simulink model "AMPC_OA_model"  (R2023b)
settings: Solver=FixedStepAuto  StartTime=0.0  StopTime=600  FixedStep=0.1  RelTol=1e-3
InitFcn:
  | clear
  | v_x = 0; v_h = 0;
  | ts = 0.1; m = 240; rou = 1.225; Cd = 1; Fx = 2.11; Fh = 1.47;
  | Kp1 = 416.55; Kp2 = 1559.85;
  | Ki1 = 133.89; Ki2 = 943.53;
  | Kd1 = 43.47; Kd2 = -103.95;
  | a1 = -0.5/m*rou*Cd*Fx*v_x; a2 = -0.5/m*rou*Cd*Fh*v_h;
  | b1 = 1/m; b2 = 1/m;
  | num = {[Kd1*b1 Kp1*b1 Ki1*b1] 0; 0 [Kd2*b2, Kp2*b2, Ki2*b2]};
  | den = {[Kd1*b1+1 Kp1*b1-a1 Ki1*b1 0] 1; 1 [Kd2*b2+1 Kp2*b2-a2 Ki2*b2 0]};
  | 
  | plant = ss(c2d(tf(num, den),ts));
  | MV = struct("Min",{0; -5},"Max",{30; 8},"RateMin",{-8*ts; -5*ts},"RateMax",{8*ts; 5*ts});
  | Weights = struct('MV',[10 10],'MVRate',[100 100],'Output',[1 1],"ECR",100000);
  | mpcobj =  mpc(plant,ts,20,1,Weights,MV);
  | E = [0 0]; F = [1 -1]; G = 0; S = 0;
  | setconstraint(mpcobj,E,F,G)
  | display(mpcobj)
  | display(tf(num, den))
StopFcn:
  | hold on
  | plot(out.x,out.h,LineWidth=2)
  | plot(polyshape([0 300 10000-300 10000],[0 300 300 0]))
libraries: slpidlib x2, mpclib x1, matrix_library x1
settings Model: Creator=Felix_Soong  LastModifiedBy=Felix_Soong

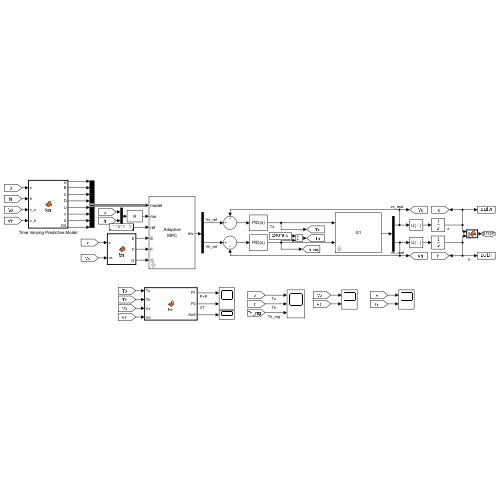
[thumbnail: Simulink's stored preview of the top-level diagram]
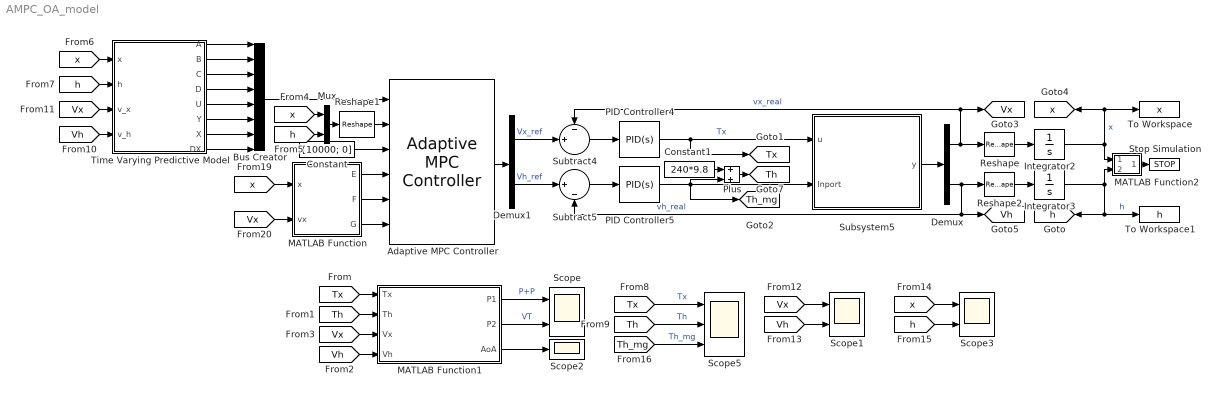
== system AMPC_OA_model ==
  Adaptive MPC Controller : mpclib/Adaptive MPC Controller  SCDEnableBlockLinearizationSpecification=on  mpcobj=mpcobj  enable_value=0  updateMPCinCallerWorkspace=on  md_inport=off  mv_inport=off  uref_inport=off  return_cost=off  return_mvseq=off  return_qpstatus=off  return_xseq=off  return_state=off  return_ovseq=off  state_inport=off  isltv_plant=off  umin_inport=off  umax_inport=off  ymin_inport=off  ymax_inport=off  cc_inport=on  ywt_inport=off  uwt_inport=off  duwt_inport=off  rhoeps_inport=off  pm_inport=off  MaximumP=10  HorizonChoice=FixedHorizon  BlockDataType=double  SampleTimeInherited=off  switch_inport=off
  Bus Creator : BusCreator  Inputs=8
  Constant : Constant  Value=[10000; 0]
  Constant1 : Constant  Value=240*9.8
  Demux : Demux  Outputs=2
  Demux1 : Demux  Outputs=2
  Integrator2 : Integrator
  Integrator3 : Integrator
  MATLAB Function : MATLAB Function  TreatAsAtomicUnit=on
  MATLAB Function1 : MATLAB Function  TreatAsAtomicUnit=on
  MATLAB Function2 : MATLAB Function  TreatAsAtomicUnit=on
  Mux : Mux  Inputs=2
  PID Controller4 : slpidlib/PID Controller  Controller=PID  Form=Parallel  TimeDomain=Continuous-time  UseExternalTs=off  SampleTime=-1  IntegratorMethod=Forward Euler  FilterMethod=Forward Euler  ControllerParametersSource=internal  P=416.552891741816  I=133.885986163438  UseKiTs=off  D=43.4731448254193  N=6.63612888550275  UseFilter=on  TunerSelectOption=Transfer Function Based (PID Tuner App)  InitialConditionSource=internal  InitialConditionForIntegrator=0  InitialConditionForFilter=0  DifferentiatorICPrevScaledInput=0  ExternalReset=none  TrackingMode=off  Kt=1  LimitOutput=off  SatLimitsSource=internal  UpperSaturationLimit=inf  LowerSaturationLimit=-inf  LinearizeAsGain=on  AntiWindupMode=none  Kb=1  LimitIntegrator=off  UpperIntegratorSaturationLimit=inf  LowerIntegratorSaturationLimit=-inf  POutMin=[]  POutMax=[]  IOutMin=[]  IOutMax=[]  DOutMin=[]  DOutMax=[]  NOutMin=[]  NOutMax=[]  SumOutMin=[]  SumOutMax=[]  SaturationOutMin=[]  SaturationOutMax=[]  PParamMin=[]  PParamMax=[]  IParamMin=[]  IParamMax=[]  DParamMin=[]  DParamMax=[]  NParamMin=[]  NParamMax=[]  KbParamMin=[]  KbParamMax=[]  KtParamMin=[]  KtParamMax=[]  KbOutMin=[]  KbOutMax=[]  KtOutMin=[]  KtOutMax=[]  IntegratorOutMin=[]  IntegratorOutMax=[]  FilterOutMin=[]  FilterOutMax=[]  SumI1OutMin=[]  SumI1OutMax=[]  SumI2OutMin=[]  SumI2OutMax=[]  SumI3OutMin=[]  SumI3OutMax=[]  SumI4OutMin=[]  SumI4OutMax=[]  SumDOutMin=[]  SumDOutMax=[]  DifferentiatorOutMin=[]  DifferentiatorOutMax=[]  FilterDiffOutCoefMin=[]  FilterDiffOutCoefMax=[]  ReciprocalOutMin=[]  ReciprocalOutMax=[]  SumDenOutMin=[]  SumDenOutMax=[]  SumNumOutMin=[]  SumNumOutMax=[]  DivideOutMin=[]  DivideOutMax=[]  UdiffTsProdOutMin=[]  UdiffTsProdOutMax=[]  NTsProdOutMin=[]  NTsProdOutMax=[]  UintegralTsProdOutMin=[]  UintegralTsProdOutMax=[]  UngainTsProdOutMin=[]  UngainTsProdOutMax=[]  ClampingZeroOutDataTypeStr=Inherit: Inherit via back propagation  ClampingZeroOutMin=[]  ClampingZeroOutMax=[]  FilterDenConstantOutDataTypeStr=Inherit: Inherit via back propagation  FilterDenConstantOutMin=[]  FilterDenConstantOutMax=[]  PCopyOutDataTypeStr=Inherit: Inherit via back propagation  PCopyOutMin=[]  PCopyOutMax=[]  NCopyOutDataTypeStr=Inherit: Inherit via back propagation  NCopyOutMin=[]  NCopyOutMax=[]  IntegratorContinuousStateAttributes=''  IntegratorStateMustResolveToSignalObject=off  IntegratorRTWStateStorageClass=Auto  FilterContinuousStateAttributes=''  FilterStateMustResolveToSignalObject=off  FilterRTWStateStorageClass=Auto  ParallelPVariant=InternalParameters  IdealPVariant=Disabled  IVariant=InternalParameters  DVariant=InternalParameters  IntegratorVariant=Continuous  SatVariant=Disabled  AWVariant=Passthrough  PCopyVariant=Disabled  TRVariant=Disabled  FdbkBlocksVariant=Forward  IdealPFdbkVariant=Disabled  SatFdbkVariant=Disabled  DerivativeFilterVariant=ContFilter  NVariant=InternalParameters  NCopyVariant=Disabled  FilterICVariant=InternalICsFilter  IntegratorICVariant=InternalICs  ExternalResetVariant=Disabled  TRSumVariant=Passthrough  SumFdbkVariant=Disabled  SumVariant=Sum_PID  TsampFilterVariant=InternalTs  TsampNgainVariant=Passthrough  TsampIntegralVariant=Disabled_SignalSpec  ExternalSaturationOutDataTypeStr=Inherit: Same as second input
  PID Controller5 : slpidlib/PID Controller  Controller=PID  Form=Parallel  TimeDomain=Continuous-time  UseExternalTs=off  SampleTime=-1  IntegratorMethod=Forward Euler  FilterMethod=Forward Euler  ControllerParametersSource=internal  P=1559.8476067563  I=943.53288128348  UseKiTs=off  D=-103.949358808692  N=5.44051767311659  UseFilter=on  TunerSelectOption=Transfer Function Based (PID Tuner App)  InitialConditionSource=internal  InitialConditionForIntegrator=0  InitialConditionForFilter=0  DifferentiatorICPrevScaledInput=0  ExternalReset=none  TrackingMode=off  Kt=1  LimitOutput=off  SatLimitsSource=internal  UpperSaturationLimit=inf  LowerSaturationLimit=-inf  LinearizeAsGain=on  AntiWindupMode=none  Kb=1  LimitIntegrator=off  UpperIntegratorSaturationLimit=inf  LowerIntegratorSaturationLimit=-inf  POutMin=[]  POutMax=[]  IOutMin=[]  IOutMax=[]  DOutMin=[]  DOutMax=[]  NOutMin=[]  NOutMax=[]  SumOutMin=[]  SumOutMax=[]  SaturationOutMin=[]  SaturationOutMax=[]  PParamMin=[]  PParamMax=[]  IParamMin=[]  IParamMax=[]  DParamMin=[]  DParamMax=[]  NParamMin=[]  NParamMax=[]  KbParamMin=[]  KbParamMax=[]  KtParamMin=[]  KtParamMax=[]  KbOutMin=[]  KbOutMax=[]  KtOutMin=[]  KtOutMax=[]  IntegratorOutMin=[]  IntegratorOutMax=[]  FilterOutMin=[]  FilterOutMax=[]  SumI1OutMin=[]  SumI1OutMax=[]  SumI2OutMin=[]  SumI2OutMax=[]  SumI3OutMin=[]  SumI3OutMax=[]  SumI4OutMin=[]  SumI4OutMax=[]  SumDOutMin=[]  SumDOutMax=[]  DifferentiatorOutMin=[]  DifferentiatorOutMax=[]  FilterDiffOutCoefMin=[]  FilterDiffOutCoefMax=[]  ReciprocalOutMin=[]  ReciprocalOutMax=[]  SumDenOutMin=[]  SumDenOutMax=[]  SumNumOutMin=[]  SumNumOutMax=[]  DivideOutMin=[]  DivideOutMax=[]  UdiffTsProdOutMin=[]  UdiffTsProdOutMax=[]  NTsProdOutMin=[]  NTsProdOutMax=[]  UintegralTsProdOutMin=[]  UintegralTsProdOutMax=[]  UngainTsProdOutMin=[]  UngainTsProdOutMax=[]  ClampingZeroOutDataTypeStr=Inherit: Inherit via back propagation  ClampingZeroOutMin=[]  ClampingZeroOutMax=[]  FilterDenConstantOutDataTypeStr=Inherit: Inherit via back propagation  FilterDenConstantOutMin=[]  FilterDenConstantOutMax=[]  PCopyOutDataTypeStr=Inherit: Inherit via back propagation  PCopyOutMin=[]  PCopyOutMax=[]  NCopyOutDataTypeStr=Inherit: Inherit via back propagation  NCopyOutMin=[]  NCopyOutMax=[]  IntegratorContinuousStateAttributes=''  IntegratorStateMustResolveToSignalObject=off  IntegratorRTWStateStorageClass=Auto  FilterContinuousStateAttributes=''  FilterStateMustResolveToSignalObject=off  FilterRTWStateStorageClass=Auto  ParallelPVariant=InternalParameters  IdealPVariant=Disabled  IVariant=InternalParameters  DVariant=InternalParameters  IntegratorVariant=Continuous  SatVariant=Disabled  AWVariant=Passthrough  PCopyVariant=Disabled  TRVariant=Disabled  FdbkBlocksVariant=Forward  IdealPFdbkVariant=Disabled  SatFdbkVariant=Disabled  DerivativeFilterVariant=ContFilter  NVariant=InternalParameters  NCopyVariant=Disabled  FilterICVariant=InternalICsFilter  IntegratorICVariant=InternalICs  ExternalResetVariant=Disabled  TRSumVariant=Passthrough  SumFdbkVariant=Disabled  SumVariant=Sum_PID  TsampFilterVariant=InternalTs  TsampNgainVariant=Passthrough  TsampIntegralVariant=Disabled_SignalSpec  ExternalSaturationOutDataTypeStr=Inherit: Same as second input
  Plus : Sum
  Reshape : Reshape
  Reshape1 : Reshape  OutputDimensionality=Customize  OutputDimensions=[2,1]
  Reshape2 : Reshape
  Scope : Scope  NumInputPorts=2
  Scope1 : Scope  NumInputPorts=2
  Scope2 : Scope
  Scope3 : Scope  NumInputPorts=2
  Scope5 : Scope  NumInputPorts=3
  Stop Simulation : Stop
  Subsystem5 : Subsystem  mask{m=240, Fx=2.11, Fh=1.47, Cd=1, rou=1.225}
      mask prompts: m "mass"; rou "air density"
      mask DialogControl ParameterGroupVar Prompt: 参数
      mask Display: disp('G1');
  Subtract4 : Sum  Inputs=-|+||
  Subtract5 : Sum  Inputs=||+|-
  Time Varying Predictive Model : MATLAB Function  TreatAsAtomicUnit=on
  To Workspace : ToWorkspace  VariableName=x  SampleTime=-1
  To Workspace1 : ToWorkspace  VariableName=h  SampleTime=-1
  tag scope: Th=global, Th_mg=global, Tx=global, Vh=global, Vx=global, h=global, x=global
  wires:
  Subtract5/1 -> PID Controller5/1
  Subtract4/1 -> PID Controller4/1
  Subsystem5/1(y) -> Demux/1
  Demux/1 -> Subtract4/1, [Vx], Reshape/1  "vx_real"
  Demux/2 -> Reshape2/1, [Vh], Subtract5/2  "vh_real"
  Integrator3/1 -> MATLAB Function2/2(h), To Workspace1/1, [h]  "h"
  Integrator2/1 -> MATLAB Function2/1(x), To Workspace/1, [x]  "x"
  PID Controller4/1 -> [Tx], Subsystem5/1(u)  "Tx"
  [Tx] -> MATLAB Function1/1(Tx)
  [Th] -> MATLAB Function1/2(Th)
  [Vx] -> MATLAB Function1/3(Vx)
  [Vh] -> MATLAB Function1/4(Vh)
  MATLAB Function1/1(P1) -> Scope/1  "P+P"
  MATLAB Function1/2(P2) -> Scope/2  "VT"
  MATLAB Function1/3(AoA) -> Scope2/1
  [Tx] -> Scope5/1  "Tx"
  [Th] -> Scope5/2  "Th"
  Time Varying Predictive Model/1(A) -> Bus Creator/1
  Time Varying Predictive Model/2(B) -> Bus Creator/2
  Time Varying Predictive Model/3(C) -> Bus Creator/3
  Time Varying Predictive Model/4(D) -> Bus Creator/4
  Time Varying Predictive Model/5(U) -> Bus Creator/5
  Time Varying Predictive Model/6(Y) -> Bus Creator/6
  Time Varying Predictive Model/7(X) -> Bus Creator/7
  Adaptive MPC Controller/1 -> Demux1/1
  Demux1/2 -> Subtract5/1  "Vh_ref"
  Demux1/1 -> Subtract4/2  "Vx_ref"
  Mux/1 -> Reshape1/1
  [x] -> Mux/1
  [h] -> Mux/2
  Constant/1 -> Adaptive MPC Controller/3
  [x] -> Time Varying Predictive Model/1(x)
  [h] -> Time Varying Predictive Model/2(h)
  [Vx] -> Time Varying Predictive Model/3(v_x)
  [Vh] -> Time Varying Predictive Model/4(v_h)
  Reshape1/1 -> Adaptive MPC Controller/2
  Bus Creator/1 -> Adaptive MPC Controller/1
  Time Varying Predictive Model/8(DX) -> Bus Creator/8
  [Vh] -> Scope1/2
  [Vx] -> Scope1/1
  [x] -> Scope3/1
  [h] -> Scope3/2
  PID Controller5/1 -> [Th_mg], Plus/2, Subsystem5/2(Inport)
  Plus/1 -> [Th]
  Constant1/1 -> Plus/1
  [Th_mg] -> Scope5/3  "Th_mg"
  Reshape/1 -> Integrator2/1
  Reshape2/1 -> Integrator3/1
  MATLAB Function2/1(y) -> Stop Simulation/1
  MATLAB Function/2(F) -> Adaptive MPC Controller/5
  MATLAB Function/1(E) -> Adaptive MPC Controller/4
  MATLAB Function/3(G) -> Adaptive MPC Controller/6
  [x] -> MATLAB Function/1(x)
  [Vx] -> MATLAB Function/2(vx)

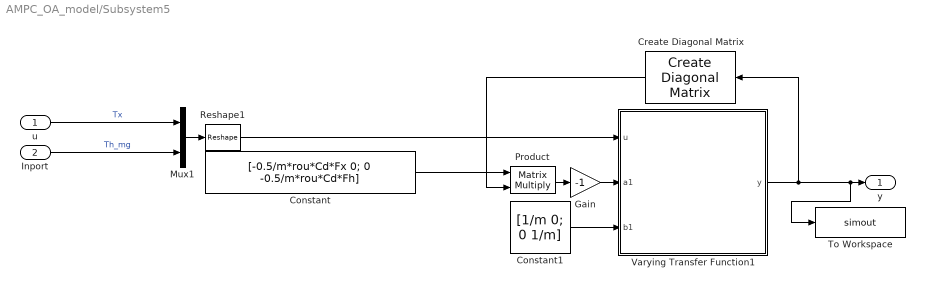
== system AMPC_OA_model/Subsystem5 ==
  u : Inport
  Inport : Inport  Port=2
  Constant : Constant  Value=[-0.5/m*rou*Cd*Fx 0; 0 -0.5/m*rou*Cd*Fh]  VectorParams1D=off
  Constant1 : Constant  Value=[1/m 0; 0 1/m]  VectorParams1D=off
  Create Diagonal Matrix : matrix_library/Create Diagonal Matrix
      settings: LibrarySourceBlock=|
      | simulink/Matrix
      | Operations/Create Diagonal
      | Matrix
  Gain : Gain  Gain=-1
  Mux1 : Mux  Inputs=2
  Product : Product  Multiplication=Matrix(*)
  Reshape1 : Reshape  OutputDimensionality=Customize  OutputDimensions=[2,1]
  To Workspace : ToWorkspace  VariableName=simout  SampleTime=-1
  Varying Transfer Function1 : Subsystem  AncestorBlock=cstblocks/Linear Parameter Varying/Varying Transfer Function  mask(Varying Transfer Function){N=1, Feedthrough=off}
      mask prompts: N "Control:simulink:VaryingTFLabel1"; Feedthrough "Control:simulink:VaryingSSLabel6"
      mask help: Control:simulink:VaryingTF1
      mask init:
      | if N~=round(N)
      |    hCB = get_param(gcb,'handle');
      |    DAStudio.slerror('Control:simulink:InvalidOrder',hCB)
      | end
      | Ts = 0;
      | SimStatus = get_param(bdroot,'SimulationStatus');
      | if any(strcmp(SimStatus,{'initializing','updating','stopped'}))
      |    controllib.internal.blocks.varying.varyingTF(gcb,N,Ts,Feedthrough)
      | end
      mask Help: eval('helpview(''control'',''VaryingTFCT'');')
      mask DialogControl N Prompt: 传递函数阶:
      mask DialogControl Feedthrough Prompt: 启用馈通
      mask Display:
      | port_label('input',2,'a1');
      | port_label('input',3,'b1');
      | plot([0.325 0.675],[0.5 0.5])
      | text(0.5, 0.7, 'b_1 s^{-1}' ,...
      |         'horizontalAlignment', 'center','texmode','on')
      | text(0.5, 0.3, '1 + a_1 s^{-1}' ,...
      |         'horizontalAlignment', 'center','texmode','on')
  y : Outport
  wires:
  Constant1/1 -> Varying Transfer Function1/3(b1)
  Constant/1 -> Product/1
  Create Diagonal Matrix/1 -> Product/2
  Mux1/1 -> Reshape1/1
  u/1 -> Mux1/1  "Tx"
  Reshape1/1 -> Varying Transfer Function1/1(u)
  Product/1 -> Gain/1
  Gain/1 -> Varying Transfer Function1/2(a1)
  Inport/1 -> Mux1/2  "Th_mg"
  Varying Transfer Function1/1(y) -> To Workspace/1, y/1, Create Diagonal Matrix/1

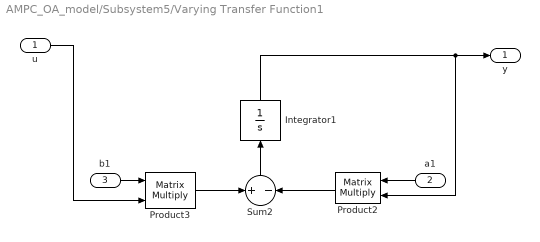
== system AMPC_OA_model/Subsystem5/Varying Transfer Function1 ==
  u : Inport
  a1 : Inport  Port=2
  b1 : Inport  Port=3
  Integrator1 : Integrator
  Product2 : Product  Multiplication=Matrix(*)  InputSameDT=on  RndMeth=Zero  SaturateOnIntegerOverflow=on  OutDataTypeStr=Inherit: Same as first input
  Product3 : Product  Multiplication=Matrix(*)  InputSameDT=on  RndMeth=Zero  SaturateOnIntegerOverflow=on  OutDataTypeStr=Inherit: Same as first input
  Sum2 : Sum  Inputs=+|-  InputSameDT=on  SaturateOnIntegerOverflow=on  OutDataTypeStr=Inherit: Same as first input
  y : Outport  VectorParamsAs1DForOutWhenUnconnected=off
  wires:
  Integrator1/1 -> Product2/2, y/1
  Sum2/1 -> Integrator1/1
  Product3/1 -> Sum2/1
  Product2/1 -> Sum2/2
  b1/1 -> Product3/1
  u/1 -> Product3/2
  a1/1 -> Product2/1

== matlab function AMPC_OA_model/MATLAB Function1 ==
  data: Tx input; P1 output; Th input; Vx input; Vh input; P2 output; AoA output
function [P1, P2, AoA] = fcn(Tx, Th, Vx, Vh)
T = sqrt(Tx^2+Th^2);
V = sqrt(Vx^2+Vh^2);

if Th ~= 0
    theta = atan(Tx/Th);
else
    theta = pi/2;
end

if Vx ~= 0
    gamma = atan(Vh/Vx);
else
    gamma = pi/2;
end

alpha = theta + gamma;
AoA = rad2deg(alpha);

A = 1.6^2 * 3.14;
P1 = T*sqrt(T/(2*1.225*A)) + T*V*sin(alpha);
P2 = T*V;

== matlab function AMPC_OA_model/MATLAB Function ==
  data: x input; E output size=[1,2]; F output size=[1,2]; vx input; G output
function [E, F, G] = fcn(x, vx)
ts = 0.1;
x_pre = x + vx * ts * 1;
if x_pre < 300
    E = [0 0]; F = [1 -1]; G = 0;
elseif x_pre >= 300 && x_pre < 10000 - 300
    E = [0 0]; F = [0 -1]; G = -300;
else
    E = [0 0]; F = [-1 -1]; G = 2 * 300 + 10000;
end

== matlab function AMPC_OA_model/MATLAB Function2 ==
  data: x input; y output; h input
function y = fcn(x, h)
if (x - 10000)^2 <= 1 && (h - 0)^2 <= 1
    y = 1;
else
    y = 0;
end

== matlab function AMPC_OA_model/Time Varying Predictive Model ==
  data: x input; h input; A output size=[6,6]; B output size=[6,2]; C output size=[2,6]; D output size=[2,2]; U output size=[2,1]; Y output size=[2,1]; X output size=[6,1]; DX output size=[6,1]; v_x input; v_h input
function [A,B,C,D,U,Y,X,DX] = fcn(x, h, v_x, v_h)
%#codegen
coder.extrinsic('ss');
coder.extrinsic('c2d');
coder.extrinsic('tf');
coder.extrinsic('ssdata');

%% constants
nx = 6;
nu = 2;
A=zeros(nx,nx);
B=zeros(nx,nu);
C=zeros(nu,nx);
D=zeros(nu,nu);

ts = 1; m = 240; rou = 1.225; Cd = 1; Fx = 2.11; Fh = 1.47;
Kp1 = 416.55; Kp2 = 1559.85;
Ki1 = 133.89; Ki2 = 943.53;
Kd1 = 43.47; Kd2 = -103.95;
a1 = -0.5/m*rou*Cd*Fx*v_x; a2 = -0.5/m*rou*Cd*Fh*v_h;
b1 = 1/m; b2 = 1/m;
num = {[Kd1*b1 Kp1*b1 Ki1*b1] 0; 0 [Kd2*b2, Kp2*b2, Ki2*b2]};
den = {[Kd1*b1+1 Kp1*b1-a1 Ki1*b1 0] 1; 1 [Kd2*b2+1 Kp2*b2-a2 Ki2*b2 0]};

%% matrix
[A,B,C,D] = ssdata(ss(c2d(tf(num, den),ts)));
%%

U = zeros(nu,1);
Y = zeros(nu,1);
X = ones(nx,1);
DX = zeros(nx,1,1);
end
